simulink model "gmskvsmsk"  (Simulink 6.0)
settings: Solver=ode45  StartTime=0.0  StopTime=Inf  RelTol=1e-3
undefined symbols (not defined in the file or in its folder): slcm
libraries: commsink2 x4, commchan2 x2, commdigbbndcpm2 x2, commrandsrc2 x1, commutil2 x1
CloseFcn:
  | clear gmskSigsOut
settings Model: Creator=mclune  LastModifiedBy=fwei  BufferReuse=off
settings DataIOCC: LimitDataPoints=off  SaveOutput=off  SaveTime=off  SignalLoggingName=gmskSigsOut
settings OptimizationCC: BooleanDataType=off  OptimizeBlockIOStorage=off  BufferReuse=off  LocalBlockOutputs=off
settings DebuggingCC: CheckExecutionContextPreStartOutputMsg=on  CheckExecutionContextRuntimeOutputMsg=on  SolverPrmCheckMsg=none
settings HardwareCC: TargetUnknown=on
settings ModelReferenceCC: UpdateModelReferenceTargets=IfOutOfDate
settings CodeAppCC: MangleLength=5
settings GRTTargetCC: LifeSpan=inf
settings SFSimCC: SFSimApplyToAllLibs=on  SFSimBuildMode=Incremental

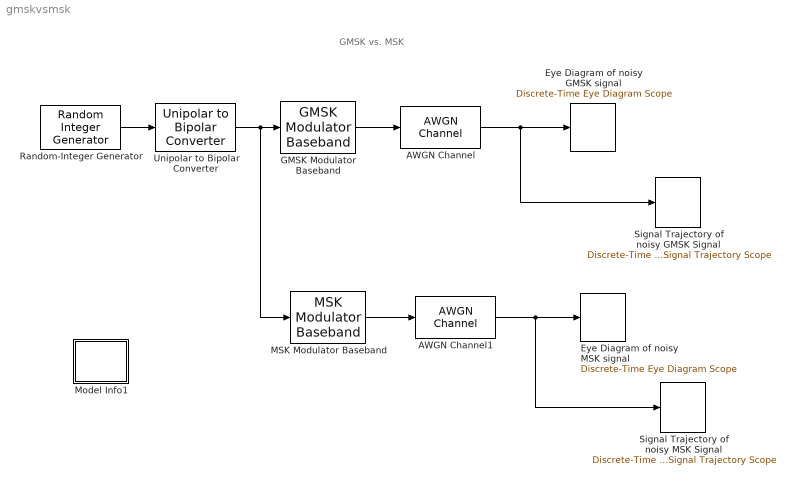
== system gmskvsmsk ==
  note: GMSK vs. MSK
  AWGN Channel : commchan2/AWGN Channel  seed=1237  noiseMode="Signal to noise ratio  (SNR)"  EbNodB=10  EsNodB=10  SNRdB=30  bitsPerSym=1  Ps=1  Tsym=1  variance=1
  AWGN Channel1 : commchan2/AWGN Channel  seed=1237  noiseMode="Signal to noise ratio  (SNR)"  EbNodB=10  EsNodB=10  SNRdB=30  bitsPerSym=1  Ps=1  Tsym=1  variance=1
  Eye Diagram of noisy GMSK signal : commsink2/Discrete-Time Eye Diagram Scope  Tag=EyeDiagram  sampPerSymb=8  offsetEye=0  symbPerTrace=2  numTraces=40  numNewFrames=10  LineStyles=-  LineColors=b  dupPoints=on  fading=on  render=on  AxisGrid=on  yMin=-1.5  yMax=1.5  inphaseLabel=In-phase Amplitude  quadratureLabel=Quadrature Amplitude  openScopeAtSimStart=on  dispDiagram=In-phase and Quadrature  FrameNumber=off  FigPos=[478 366 307 353]  figTitle=Eye Diagram  block_type_=eye  numLinesMax=8
  Eye Diagram of noisy MSK signal : commsink2/Discrete-Time Eye Diagram Scope  Tag=EyeDiagram  sampPerSymb=8  offsetEye=0  symbPerTrace=2  numTraces=40  numNewFrames=10  LineStyles=-  LineColors=m  dupPoints=on  fading=on  render=on  AxisGrid=on  yMin=-1.5  yMax=1.5  inphaseLabel=In-phase Amplitude  quadratureLabel=Quadrature Amplitude  openScopeAtSimStart=on  dispDiagram=In-phase and Quadrature  FrameNumber=off  FigPos=[161 365 307 353]  figTitle=Eye Diagram  block_type_=eye  numLinesMax=8
  GMSK Modulator Baseband : commdigbbndcpm2/GMSK Modulator Baseband  inputType=Integer  BT=.3  pulseLength=3  preHistory=1  phaseOffset=0  samplesPerSymbol=8
  MSK Modulator Baseband : commdigbbndcpm2/MSK Modulator Baseband  inputType=Integer  phaseOffset=0  samplesPerSymbol=8
  Model Info1 : Subsystem  LoadFcn=slcm LoadBlock;  InitFcn=slcm('UpdateAllCMBlocksInThisModelInit')  EnableExecutionContextPropagation=on  mask(CMBlock){InitialSaveTempField=, InitialBlockCM=None, BlockCM=None, Frame=on, SaveTempField=, DisplayStringWithTags=Info, MaskDisplayString=Info, HorizontalTextAlignment=Center, LeftAlignmentValue=0.5, SourceBlockDiagram=gmskvsmsk, TagMaxNumber=20, CMTag1=, CMTag2=, CMTag3=, CMTag4=, CMTag5=, CMTag6=, CMTag7=, CMTag8=, CMTag9=, CMTag10=, CMTag11=, CMTag12=, CMTag13=, CMTag14=, CMTag15=, CMTag16=, CMTag17=, CMTag18=, CMTag19=, CMTag20=}
      mask help: This block allows revision control information to be displayed within the model.
      settings: CopyFcn=slcm CopyBlock;  DeleteFcn=slcm Cancel;  PostSaveFcn=slcm('UpdateAllCMBlocksInThisModel')  NameChangeFcn=slcm Rename;  OpenFcn=commdemohelp;
      mask Display: text(str2num(LeftAlignmentValue), 0.5, MaskDisplayString, 'HorizontalAlignment', HorizontalTextAlignment)
  Random-Integer Generator : commrandsrc2/Random Integer Generator  mul=2  seed=[12345]  Ts=1  frameBased=on  sampPerFrame=50  orient=off
  Signal Trajectory of noisy GMSK Signal : commsink2/Discrete-Time Signal Trajectory Scope  Tag=SignalTrajectory  sampPerSymb=8  offsetEye=0  numTraces=40  numNewFrames=10  LineStyles=-  LineColors=b  fading=on  render=on  AxisGrid=on  xMin=-1.25  xMax=1.25  yMin=-1.25  yMax=1.25  inphaseLabel=In-phase Amplitude  quadratureLabel=Quadrature Amplitude  openScopeAtSimStart=off  FrameNumber=off  FigPos=[606 34 338 338]  figTitle=Signal Trajectory  numLinesMax=8  block_type_=xy
  Signal Trajectory of noisy MSK Signal : commsink2/Discrete-Time Signal Trajectory Scope  Tag=SignalTrajectory  sampPerSymb=8  offsetEye=0  numTraces=40  numNewFrames=10  LineStyles=-  LineColors=m  fading=on  render=on  AxisGrid=on  xMin=-1.25  xMax=1.25  yMin=-1.25  yMax=1.25  inphaseLabel=In-phase Amplitude  quadratureLabel=Quadrature Amplitude  openScopeAtSimStart=off  FrameNumber=off  FigPos=[257 34 338 338]  figTitle=Signal Trajectory  numLinesMax=8  block_type_=xy
  Unipolar to Bipolar Converter : commutil2/Unipolar to Bipolar Converter  M=2  polarity=Positive
  wires:
  Random-Integer Generator/1 -> Unipolar to Bipolar Converter/1
  GMSK Modulator Baseband/1 -> AWGN Channel/1
  AWGN Channel/1 -> Eye Diagram of noisy GMSK signal/1, Signal Trajectory of noisy GMSK Signal/1
  Unipolar to Bipolar Converter/1 -> GMSK Modulator Baseband/1, MSK Modulator Baseband/1
  MSK Modulator Baseband/1 -> AWGN Channel1/1
  AWGN Channel1/1 -> Eye Diagram of noisy MSK signal/1, Signal Trajectory of noisy MSK Signal/1

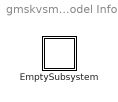
== system gmskvsmsk/Model Info1 ==
  EmptySubsystem : Subsystem  EnableExecutionContextPropagation=on

== system gmskvsmsk/Model Info1/EmptySubsystem ==
